simulink library "ADV_BF_MASTER"  (Simulink 8.6)
settings: Solver=VariableStepAuto  StartTime=0.0  StopTime=10.0  RelTol=1e-3
libraries: cdsEpicsOut x43, cdsFilt x36, cdsTP x20, cdsFiltCtrl x17, cdsEpicsIn x10, cdsMuxMatrix x4, VIS_LIB x2, cdsEpicsBinIn x2, cdsOsc x1, cdsFunctionCall x1, SIXOSEM_F_STAGE_MASTER x1
(part 1 of 6)
settings Model: Creator=controls  LastModifiedBy=controls

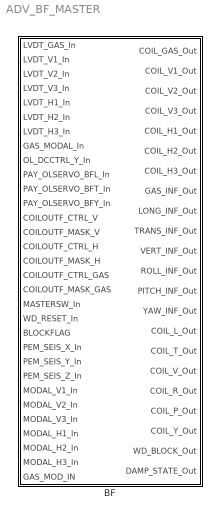
== system ADV_BF_MASTER ==
  BF : Subsystem

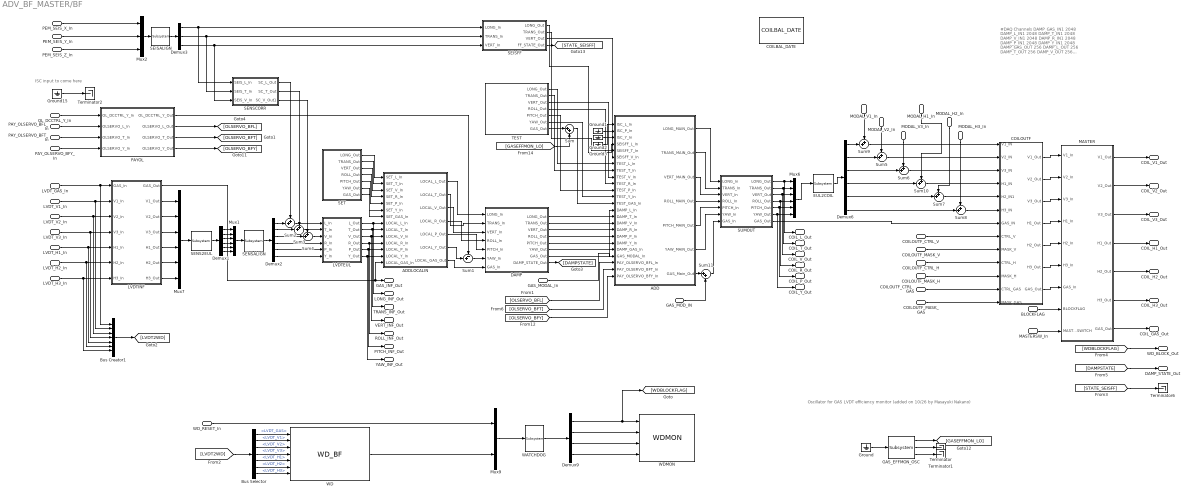
== system ADV_BF_MASTER/BF ==
  note: #DAQ Channels
      | DAMP_GAS_IN1 2048
      | DAMP_L_IN1 2048
      | DAMP_T_IN1 2048
      | DAMP_V_IN1 2048
      | DAMP_R_IN1 2048
      | DAMP_P_IN1 2048
      | DAMP_Y_IN1 2048
      | DAMP_GAS_OUT 256
      | DAMP_L_OUT 256
      | DAMP_T_OUT 256
      | DAMP_V_OUT 256
      | DAMP_R_OUT 256
      | DAMP_P_OUT 256
      | DAMP_Y_OUT 256
      | LVDTINF_GAS_IN1 2048
  note: ISC input to come here
  note: Oscillator for GAS LVDT efficiency monitor (added on 10/26 by Masayuki Nakano)
  LVDT_GAS_In : Inport
  LVDT_V1_In : Inport  Port=2
  LVDT_V2_In : Inport  Port=3
  LVDT_V3_In : Inport  Port=4
  LVDT_H1_In : Inport  Port=5
  LVDT_H2_In : Inport  Port=6
  LVDT_H3_In : Inport  Port=7
  GAS_MODAL_In : Inport  Port=8
  OL_DCCTRL_Y_In : Inport  Port=9
  PAY_OLSERVO_BFL_In : Inport  Port=10
  PAY_OLSERVO_BFT_In : Inport  Port=11
  PAY_OLSERVO_BFY_In : Inport  Port=12
  COILOUTF_CTRL_V : Inport  Port=13
  COILOUTF_MASK_V : Inport  Port=14
  COILOUTF_CTRL_H : Inport  Port=15
  COILOUTF_MASK_H : Inport  Port=16
  COILOUTF_CTRL_GAS : Inport  Port=17
  COILOUTF_MASK_GAS : Inport  Port=18
  MASTERSW_In : Inport  Port=19
  WD_RESET_In : Inport  Port=20
  BLOCKFLAG : Inport  Port=21
  PEM_SEIS_X_In : Inport  Port=22
  PEM_SEIS_Y_In : Inport  Port=23
  PEM_SEIS_Z_In : Inport  Port=24
  MODAL_V1_In : Inport  Port=25
  MODAL_V2_In : Inport  Port=26
  MODAL_V3_In : Inport  Port=27
  MODAL_H1_In : Inport  Port=28
  MODAL_H2_In : Inport  Port=29
  MODAL_H3_In : Inport  Port=30
  GAS_MOD_IN : Inport  Port=31
  ADD : Subsystem
  ADDLOCALIN : Subsystem
  Bus Creator1 : BusCreator  Inputs='LVDT_GAS','LVDT_V1','LVDT_V2','LVDT_V3','LVDT_H1','LVDT_H2','LVDT_H3'
  Bus Selector : BusSelector  OutputSignals=LVDT_GAS,LVDT_V1,LVDT_V2,LVDT_V3,LVDT_H1,LVDT_H2,LVDT_H3
  COILBAL_DATE : VIS_LIB/COILBAL_DATE
  COILOUTF : Subsystem
  DAMP : Subsystem
  Demux1 : Demux  Outputs=6
  Demux2 : Demux  Outputs=6
  Demux3 : Demux  Outputs=3
  Demux6 : Demux  Outputs=6
  Demux9 : Demux
  EUL2COIL : cdsMuxMatrix/Subsystem  Tag=cdsMuxMatrix  Description=|
      | ADL=SUS_INMATRIX.adl
      | SCRIPT=generate_KisselButton.py 4 5 #CHANNEL# > #TARGET_DIR#/#FULL_PART_NAME#_KB.adl
      settings: AttributesFormatString=%<Tag>
  GAS_EFFMON_OSC : cdsOsc/Subsystem  Tag=cdsOsc  Description=Oscillator
      settings: AttributesFormatString=%<Tag>
  Ground{,1..3,15} (5 alike) : Ground
  LVDTEUL : Subsystem
  LVDTINF : Subsystem
  MASTER : Subsystem
  Mux1 : Mux  Inputs=6
  Mux2 : Mux  Inputs=3
  Mux6 : Mux  Inputs=6
  Mux7 : Mux  Inputs=6
  Mux9 : Mux  Inputs=2
  PAYOL : Subsystem
  SEISALIGN : cdsMuxMatrix/Subsystem  Tag=cdsMuxMatrix  Description=|
      | ADL=SUS_INMATRIX.adl
      | SCRIPT=generate_KisselButton.py 4 5 #CHANNEL# > #TARGET_DIR#/#FULL_PART_NAME#_KB.adl
      settings: AttributesFormatString=%<Tag>
  SEISFF : Subsystem
  SENS2EUL : cdsMuxMatrix/Subsystem  Tag=cdsMuxMatrix  Description=Any size matrix. Inputs and outputs must be connected using Mux and Demux parts.
      settings: AttributesFormatString=%<Tag>
  SENSALIGN : cdsMuxMatrix/Subsystem  Tag=cdsMuxMatrix  Description=Any size matrix. Inputs and outputs must be connected using Mux and Demux parts.
      settings: AttributesFormatString=%<Tag>
  SENSCORR : Subsystem
  SET : Subsystem
  SUMOUT : Subsystem
  Sum : Sum  Inputs=|++
  Sum1 : Sum  Inputs=-+|
  Sum{2..10} (9 alike) : Sum  Inputs=++|
  Sum11 : Sum  Inputs=|++
  TEST : Subsystem
  Terminator{,1..2,6} (4 alike) : Terminator
  WATCHDOG : cdsFunctionCall/Subsystem  Tag=cdsFunctionCall  Description=inline OSEMWATCHDOG /opt/rtcds/userapps/release/vis/common/src/WATCHDOG.c
      settings: AttributesFormatString=%<Tag>\n%<Description>
  WD : VIS_LIB/WD_BF
  WDMON : SIXOSEM_F_STAGE_MASTER/SIXOSEM_F_STAGE_MASTER/WDMON
  COIL_GAS_Out : Outport
  COIL_V1_Out : Outport  Port=2
  COIL_V2_Out : Outport  Port=3
  COIL_V3_Out : Outport  Port=4
  COIL_H1_Out : Outport  Port=5
  COIL_H2_Out : Outport  Port=6
  COIL_H3_Out : Outport  Port=7
  GAS_INF_Out : Outport  Port=8
  LONG_INF_Out : Outport  Port=9
  TRANS_INF_Out : Outport  Port=10
  VERT_INF_Out : Outport  Port=11
  ROLL_INF_Out : Outport  Port=12
  PITCH_INF_Out : Outport  Port=13
  YAW_INF_Out : Outport  Port=14
  COIL_L_Out : Outport  Port=15
  COIL_T_Out : Outport  Port=16
  COIL_V_Out : Outport  Port=17
  COIL_R_Out : Outport  Port=18
  COIL_P_Out : Outport  Port=19
  COIL_Y_Out : Outport  Port=20
  WD_BLOCK_Out : Outport  Port=21
  DAMP_STATE_Out : Outport  Port=22
  wires:
  GAS_MOD_IN/1 -> Sum11/2
  Sum11/1 -> SUMOUT/7(GAS_In)
  ADD/7(GAS_Main_Out) -> Sum11/1
  Demux6/1 -> Sum9/2
  Demux6/6 -> Sum8/2
  MODAL_H3_In/1 -> Sum8/1
  Sum8/1 -> COILOUTF/6(H3_IN)
  Demux6/5 -> Sum7/2
  MODAL_H2_In/1 -> Sum7/1
  Sum7/1 -> COILOUTF/5(H2_IN1)
  Demux6/4 -> Sum10/2
  MODAL_H1_In/1 -> Sum10/1
  Sum10/1 -> COILOUTF/4(H1_IN)
  Demux6/3 -> Sum6/2
  MODAL_V3_In/1 -> Sum6/1
  Sum6/1 -> COILOUTF/3(V3_IN)
  Demux6/2 -> Sum5/2
  MODAL_V2_In/1 -> Sum5/1
  Sum5/1 -> COILOUTF/2(V2_IN)
  MODAL_V1_In/1 -> Sum9/1
  Sum9/1 -> COILOUTF/1(V1_IN)
  Ground15/1 -> Terminator2/1
  GAS_EFFMON_OSC/3 -> Terminator1/1
  GAS_EFFMON_OSC/2 -> Terminator/1
  Ground/1 -> GAS_EFFMON_OSC/1
  [GASEFFMON_LO] -> Sum/2
  TEST/7(GAS_Out) -> Sum/1
  GAS_EFFMON_OSC/1 -> [GASEFFMON_LO]
  COILOUTF_MASK_GAS/1 -> COILOUTF/13(MASK_GAS)
  COILOUTF_CTRL_GAS/1 -> COILOUTF/12(CTRL_GAS)
  COILOUTF_MASK_H/1 -> COILOUTF/11(MASK_H)
  COILOUTF_CTRL_H/1 -> COILOUTF/10(CTRL_H)
  LVDTINF/7(H3_Out) -> Mux7/6
  LVDTINF/6(H2_Out) -> Mux7/5
  LVDTINF/5(H1_Out) -> Mux7/4
  Bus Selector/7 -> WD/7  "<LVDT_H3>"
  Bus Selector/6 -> WD/6  "<LVDT_H2>"
  Bus Selector/5 -> WD/5  "<LVDT_H1>"
  Bus Selector/4 -> WD/4  "<LVDT_V3>"
  Bus Selector/3 -> WD/3  "<LVDT_V2>"
  Bus Selector/2 -> WD/2  "<LVDT_V1>"
  [DAMPSTATE] -> DAMP_STATE_Out/1
  [WDBLOCKFLAG] -> WD_BLOCK_Out/1
  MASTER/7(GAS_Out) -> COIL_GAS_Out/1
  MASTER/6(H3_Out) -> COIL_H3_Out/1
  MASTER/5(H2_Out) -> COIL_H2_Out/1
  MASTERSW_In/1 -> MASTER/9(MASTERSWITCH)
  BLOCKFLAG/1 -> MASTER/8(BLOCKFLAG)
  COILOUTF/4(H1_Out) -> MASTER/4(H1_In)
  COILOUTF/3(V3_Out) -> MASTER/3(V3_In)
  COILOUTF/2(V2_Out) -> MASTER/2(V2_In)
  COILOUTF/1(V1_Out) -> MASTER/1(V1_In)
  COILOUTF/7(GAS_Out) -> MASTER/7(GAS_In)
  COILOUTF/6(H3_Out) -> MASTER/6(H3_In)
  COILOUTF/5(H2_Out) -> MASTER/5(H2_In)
  DAMP/1(LONG_Out) -> ADD/14(DAMP_L_In)
  DAMP/2(TRANS_Out) -> ADD/15(DAMP_T_In)
  DAMP/3(VERT_Out) -> ADD/16(DAMP_V_In)
  DAMP/4(ROLL_Out) -> ADD/17(DAMP_R_In)
  DAMP/5(PITCH_Out) -> ADD/18(DAMP_P_In)
  DAMP/6(YAW_Out) -> ADD/19(DAMP_Y_In)
  DAMP/7(GAS_Out) -> ADD/20(DAMP_GAS_In)
  DAMP/8(DAMP_STATE_Out) -> [DAMPSTATE]
  LVDTINF/4(V3_Out) -> Mux7/3
  LVDTINF/3(V2_Out) -> Mux7/2
  LVDTINF/2(V1_Out) -> Mux7/1
  SENSALIGN/1 -> Demux2/1
  Mux1/1 -> SENSALIGN/1
  Demux1/6 -> Mux1/6
  Demux1/5 -> Mux1/5
  Demux1/4 -> Mux1/4
  Demux1/3 -> Mux1/3
  Demux1/2 -> Mux1/2
  Demux1/1 -> Mux1/1
  SENS2EUL/1 -> Demux1/1
  Bus Selector/1 -> WD/1  "<LVDT_GAS>"
  MASTER/4(H1_Out) -> COIL_H1_Out/1
  LVDT_GAS_In/1 -> LVDTINF/1(GAS_In), Bus Creator1/1
  COILOUTF_MASK_V/1 -> COILOUTF/9(MASK_V)
  COILOUTF_CTRL_V/1 -> COILOUTF/8(CTRL_V)
  Bus Creator1/1 -> [LVDT2WD]
  LVDT_H3_In/1 -> Bus Creator1/7, LVDTINF/7(H3_In)
  LVDT_H2_In/1 -> Bus Creator1/6, LVDTINF/6(H2_In)
  LVDT_H1_In/1 -> Bus Creator1/5, LVDTINF/5(H1_In)
  LVDT_V3_In/1 -> LVDTINF/4(V3_In), Bus Creator1/4
  LVDT_V2_In/1 -> LVDTINF/3(V2_In), Bus Creator1/3
  LVDT_V1_In/1 -> LVDTINF/2(V1_In), Bus Creator1/2
  WATCHDOG/1 -> Demux9/1
  Mux9/1 -> WATCHDOG/1
  Demux9/4 -> WDMON/4
  Demux9/3 -> WDMON/3
  Demux9/2 -> WDMON/2
  Demux9/1 -> WDMON/1, [WDBLOCKFLAG]
  [LVDT2WD] -> Bus Selector/1
  WD/1 -> Mux9/2
  WD_RESET_In/1 -> Mux9/1
  MASTER/3(V3_Out) -> COIL_V3_Out/1
  MASTER/2(V2_Out) -> COIL_V2_Out/1
  MASTER/1(V1_Out) -> COIL_V1_Out/1
  EUL2COIL/1 -> Demux6/1
  Mux6/1 -> EUL2COIL/1
  Mux7/1 -> SENS2EUL/1
  GAS_MODAL_In/1 -> ADD/21(GAS_MODAL_In)
  Ground1/1 -> ADD/1(ISC_L_In)
  Ground2/1 -> ADD/2(ISC_P_In)
  Ground3/1 -> ADD/3(ISC_Y_In)
  OL_DCCTRL_Y_In/1 -> PAYOL/1(OL_DCCTRL_Y_In)
  PAY_OLSERVO_BFY_In/1 -> PAYOL/4(OLSERVO_Y_In)
  PAYOL/4(OLSERVO_Y_Out) -> [OLSERVO_BFY]
  [OLSERVO_BFY] -> ADD/24(PAY_OLSERVO_BFY_In)
  SEISFF/4(FF_STATE_Out) -> [STATE_SEISFF]
  PEM_SEIS_Y_In/1 -> Mux2/2
  PEM_SEIS_X_In/1 -> Mux2/1
  Mux2/1 -> SEISALIGN/1
  SEISALIGN/1 -> Demux3/1
  Demux3/2 -> SEISFF/2(TRANS_In), SENSCORR/2(SEIS_T_In)
  Demux3/1 -> SEISFF/1(LONG_In), SENSCORR/1(SEIS_L_In)
  PEM_SEIS_Z_In/1 -> Mux2/3
  Demux3/3 -> SEISFF/3(VERT_In), SENSCORR/3(SEIS_V_In)
  SENSCORR/1(SC_L_Out) -> Sum2/1
  SENSCORR/2(SC_T_Out) -> Sum3/1
  SENSCORR/3(SC_V_Out1) -> Sum4/1
  Demux2/1 -> Sum2/2
  Demux2/2 -> Sum3/2
  Demux2/3 -> Sum4/2
  TEST/1(LONG_Out) -> ADD/7(TEST_L_In)
  TEST/2(TRANS_Out) -> ADD/8(TEST_T_In)
  TEST/3(VERT_Out) -> ADD/9(TEST_V_In)
  TEST/4(ROLL_Out) -> ADD/10(TEST_R_In)
  TEST/5(PITCH_Out) -> ADD/11(TEST_P_In)
  TEST/6(YAW_Out) -> ADD/12(TEST_Y_In)
  Sum/1 -> ADD/13(TEST_GAS_In)
  [STATE_SEISFF] -> Terminator6/1
  SEISFF/3(VERT_Out) -> ADD/6(SEISFF_V_In)
  SEISFF/1(LONG_Out) -> ADD/4(SEISFF_L_In)
  SEISFF/2(TRANS_Out) -> ADD/5(SEISFF_T_In)
  Sum2/1 -> LVDTEUL/1(L_In)
  Sum3/1 -> LVDTEUL/2(T_In)
  Sum4/1 -> LVDTEUL/3(V_In)
  Demux2/4 -> LVDTEUL/4(R_In)
  Demux2/5 -> LVDTEUL/5(P_In)
  Demux2/6 -> LVDTEUL/6(Y_In)
  SET/2(TRANS_Out) -> ADDLOCALIN/2(SET_T_In)
  SET/3(VERT_Out) -> ADDLOCALIN/3(SET_V_In)
  SET/7(GAS_Out) -> ADDLOCALIN/7(SET_GAS_In)
  SET/5(PITCH_Out) -> ADDLOCALIN/5(SET_P_In)
  SET/1(LONG_Out) -> ADDLOCALIN/1(SET_L_In)
  SET/4(ROLL_Out) -> ADDLOCALIN/4(SET_R_In)
  SET/6(YAW_Out) -> ADDLOCALIN/6(SET_Y_In)
  LVDTEUL/6(Y_Out) -> YAW_INF_Out/1, ADDLOCALIN/13(LOCAL_Y_In)
  LVDTEUL/1(L_Out) -> LONG_INF_Out/1, ADDLOCALIN/8(LOCAL_L_In)
  LVDTEUL/2(T_Out) -> TRANS_INF_Out/1, ADDLOCALIN/9(LOCAL_T_In)
  LVDTEUL/3(V_Out) -> VERT_INF_Out/1, ADDLOCALIN/10(LOCAL_V_In)
  LVDTEUL/4(R_Out) -> ROLL_INF_Out/1, ADDLOCALIN/11(LOCAL_R_In)
  LVDTEUL/5(P_Out) -> PITCH_INF_Out/1, ADDLOCALIN/12(LOCAL_P_In)
  ADDLOCALIN/7(LOCAL_GAS_Out) -> DAMP/7(GAS_In)
  ADDLOCALIN/6(LOCAL_Y_Out) -> Sum1/2
  ADDLOCALIN/5(LOCAL_P_Out) -> DAMP/5(PITCH_In)
  ADDLOCALIN/4(LOCAL_R_Out) -> DAMP/4(ROLL_In)
  ADDLOCALIN/3(LOCAL_V_Out) -> DAMP/3(VERT_In)
  ADDLOCALIN/2(LOCAL_T_Out) -> DAMP/2(TRANS_In)
  ADDLOCALIN/1(LOCAL_L_Out) -> DAMP/1(LONG_In)
  LVDTINF/1(GAS_Out) -> GAS_INF_Out/1, ADDLOCALIN/14(LOCAL_GAS_In)
  Sum1/1 -> DAMP/6(YAW_In)
  PAYOL/1(OL_DCCTRL_Y_Out) -> Sum1/1
  [OLSERVO_BFL] -> ADD/22(PAY_OLSERVO_BFL_In)
  [OLSERVO_BFT] -> ADD/23(PAY_OLSERVO_BFT_In)
  PAY_OLSERVO_BFL_In/1 -> PAYOL/2(OLSERVO_L_In)
  PAY_OLSERVO_BFT_In/1 -> PAYOL/3(OLSERVO_T_In)
  PAYOL/3(OLSERVO_T_Out) -> [OLSERVO_BFT]
  PAYOL/2(OLSERVO_L_Out) -> [OLSERVO_BFL]
  SUMOUT/1(LONG_Out) -> COIL_L_Out/1, Mux6/1
  SUMOUT/6(YAW_Out) -> COIL_Y_Out/1, Mux6/6
  SUMOUT/3(VERT_Out) -> COIL_V_Out/1, Mux6/3
  SUMOUT/2(TRANS_Out) -> COIL_T_Out/1, Mux6/2
  SUMOUT/4(ROLL_Out) -> COIL_R_Out/1, Mux6/4
  SUMOUT/5(PITCH_Out) -> COIL_P_Out/1, Mux6/5
  SUMOUT/7(GAS_Out) -> COILOUTF/7(GAS_IN)
  ADD/4(ROLL_MAIN_Out) -> SUMOUT/4(ROLL_In)
  ADD/3(VERT_MAIN_Out) -> SUMOUT/3(VERT_In)
  ADD/5(PITCH_MAIN_Out) -> SUMOUT/5(PITCH_In)
  ADD/2(TRANS_MAIN_Out) -> SUMOUT/2(TRANS_In)
  ADD/6(YAW_MAIN_Out) -> SUMOUT/6(YAW_In)
  ADD/1(LONG_MAIN_Out) -> SUMOUT/1(LONG_In)

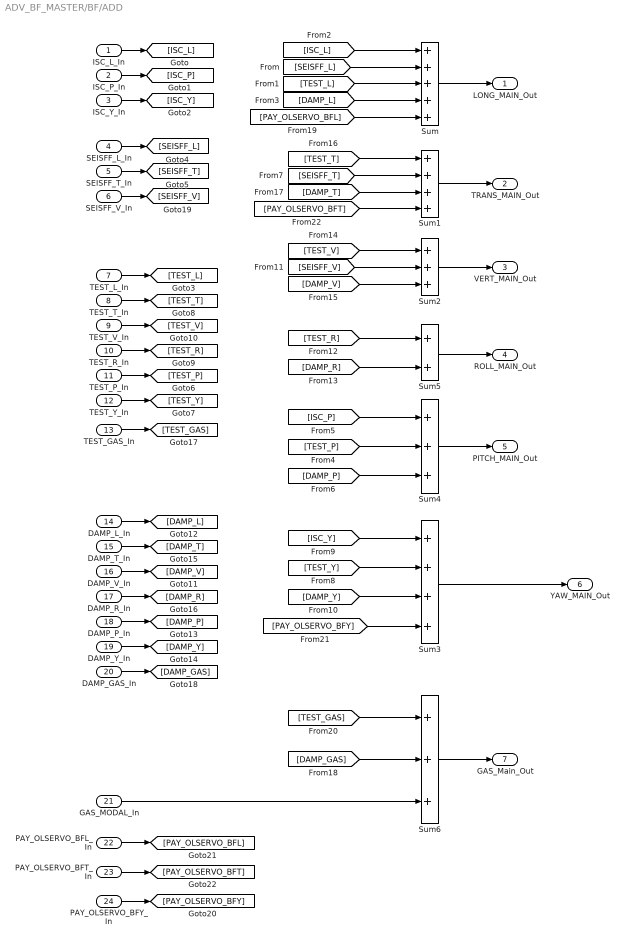
== system ADV_BF_MASTER/BF/ADD ==
  ISC_L_In : Inport
  ISC_P_In : Inport  Port=2
  ISC_Y_In : Inport  Port=3
  SEISFF_L_In : Inport  Port=4
  SEISFF_T_In : Inport  Port=5
  SEISFF_V_In : Inport  Port=6
  TEST_L_In : Inport  Port=7
  TEST_T_In : Inport  Port=8
  TEST_V_In : Inport  Port=9
  TEST_R_In : Inport  Port=10
  TEST_P_In : Inport  Port=11
  TEST_Y_In : Inport  Port=12
  TEST_GAS_In : Inport  Port=13
  DAMP_L_In : Inport  Port=14
  DAMP_T_In : Inport  Port=15
  DAMP_V_In : Inport  Port=16
  DAMP_R_In : Inport  Port=17
  DAMP_P_In : Inport  Port=18
  DAMP_Y_In : Inport  Port=19
  DAMP_GAS_In : Inport  Port=20
  GAS_MODAL_In : Inport  Port=21
  PAY_OLSERVO_BFL_In : Inport  Port=22
  PAY_OLSERVO_BFT_In : Inport  Port=23
  PAY_OLSERVO_BFY_In : Inport  Port=24
  Sum : Sum  Inputs=+++++
  Sum1 : Sum  Inputs=++++
  Sum2 : Sum  Inputs=+++
  Sum3 : Sum  Inputs=++++
  Sum4 : Sum  Inputs=+++
  Sum5 : Sum
  Sum6 : Sum  Inputs=+++
  LONG_MAIN_Out : Outport
  TRANS_MAIN_Out : Outport  Port=2
  VERT_MAIN_Out : Outport  Port=3
  ROLL_MAIN_Out : Outport  Port=4
  PITCH_MAIN_Out : Outport  Port=5
  YAW_MAIN_Out : Outport  Port=6
  GAS_Main_Out : Outport  Port=7
  wires:
  DAMP_GAS_In/1 -> [DAMP_GAS]
  DAMP_Y_In/1 -> [DAMP_Y]
  DAMP_P_In/1 -> [DAMP_P]
  DAMP_R_In/1 -> [DAMP_R]
  DAMP_V_In/1 -> [DAMP_V]
  DAMP_T_In/1 -> [DAMP_T]
  DAMP_L_In/1 -> [DAMP_L]
  TEST_GAS_In/1 -> [TEST_GAS]
  TEST_Y_In/1 -> [TEST_Y]
  TEST_P_In/1 -> [TEST_P]
  TEST_R_In/1 -> [TEST_R]
  TEST_V_In/1 -> [TEST_V]
  TEST_T_In/1 -> [TEST_T]
  TEST_L_In/1 -> [TEST_L]
  SEISFF_V_In/1 -> [SEISFF_V]
  Sum6/1 -> GAS_Main_Out/1
  Sum4/1 -> PITCH_MAIN_Out/1
  Sum/1 -> LONG_MAIN_Out/1
  [ISC_L] -> Sum/1
  [TEST_L] -> Sum/3
  [DAMP_L] -> Sum/4
  Sum5/1 -> ROLL_MAIN_Out/1
  Sum2/1 -> VERT_MAIN_Out/1
  Sum1/1 -> TRANS_MAIN_Out/1
  SEISFF_L_In/1 -> [SEISFF_L]
  SEISFF_T_In/1 -> [SEISFF_T]
  ISC_L_In/1 -> [ISC_L]
  ISC_P_In/1 -> [ISC_P]
  ISC_Y_In/1 -> [ISC_Y]
  [ISC_P] -> Sum4/1
  [TEST_R] -> Sum5/1
  [DAMP_R] -> Sum5/2
  [TEST_T] -> Sum1/1
  [DAMP_T] -> Sum1/3
  [TEST_V] -> Sum2/1
  [DAMP_V] -> Sum2/3
  PAY_OLSERVO_BFY_In/1 -> [PAY_OLSERVO_BFY]
  Sum3/1 -> YAW_MAIN_Out/1
  [SEISFF_L] -> Sum/2
  [SEISFF_T] -> Sum1/2
  [SEISFF_V] -> Sum2/2
  [TEST_P] -> Sum4/2
  [DAMP_P] -> Sum4/3
  [PAY_OLSERVO_BFY] -> Sum3/4
  [DAMP_Y] -> Sum3/3
  [TEST_Y] -> Sum3/2
  [ISC_Y] -> Sum3/1
  [TEST_GAS] -> Sum6/1
  [DAMP_GAS] -> Sum6/2
  GAS_MODAL_In/1 -> Sum6/3
  PAY_OLSERVO_BFL_In/1 -> [PAY_OLSERVO_BFL]
  PAY_OLSERVO_BFT_In/1 -> [PAY_OLSERVO_BFT]
  [PAY_OLSERVO_BFL] -> Sum/5
  [PAY_OLSERVO_BFT] -> Sum1/4

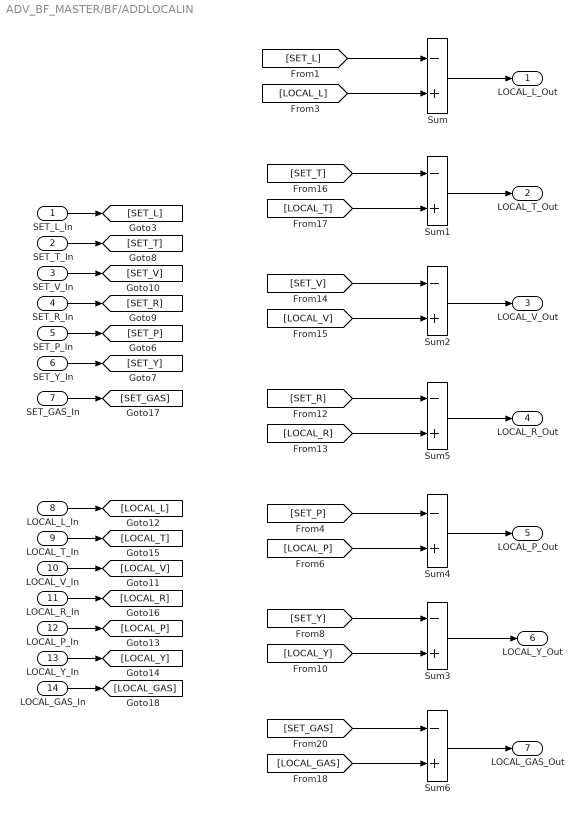
== system ADV_BF_MASTER/BF/ADDLOCALIN ==
  SET_L_In : Inport
  SET_T_In : Inport  Port=2
  SET_V_In : Inport  Port=3
  SET_R_In : Inport  Port=4
  SET_P_In : Inport  Port=5
  SET_Y_In : Inport  Port=6
  SET_GAS_In : Inport  Port=7
  LOCAL_L_In : Inport  Port=8
  LOCAL_T_In : Inport  Port=9
  LOCAL_V_In : Inport  Port=10
  LOCAL_R_In : Inport  Port=11
  LOCAL_P_In : Inport  Port=12
  LOCAL_Y_In : Inport  Port=13
  LOCAL_GAS_In : Inport  Port=14
  Sum{,1..6} (7 alike) : Sum  Inputs=-+
  LOCAL_L_Out : Outport
  LOCAL_T_Out : Outport  Port=2
  LOCAL_V_Out : Outport  Port=3
  LOCAL_R_Out : Outport  Port=4
  LOCAL_P_Out : Outport  Port=5
  LOCAL_Y_Out : Outport  Port=6
  LOCAL_GAS_Out : Outport  Port=7
  wires:
  LOCAL_GAS_In/1 -> [LOCAL_GAS]
  LOCAL_Y_In/1 -> [LOCAL_Y]
  LOCAL_P_In/1 -> [LOCAL_P]
  LOCAL_R_In/1 -> [LOCAL_R]
  LOCAL_V_In/1 -> [LOCAL_V]
  LOCAL_T_In/1 -> [LOCAL_T]
  LOCAL_L_In/1 -> [LOCAL_L]
  SET_GAS_In/1 -> [SET_GAS]
  SET_Y_In/1 -> [SET_Y]
  SET_P_In/1 -> [SET_P]
  SET_R_In/1 -> [SET_R]
  SET_V_In/1 -> [SET_V]
  SET_T_In/1 -> [SET_T]
  SET_L_In/1 -> [SET_L]
  Sum6/1 -> LOCAL_GAS_Out/1
  Sum4/1 -> LOCAL_P_Out/1
  Sum/1 -> LOCAL_L_Out/1
  Sum5/1 -> LOCAL_R_Out/1
  Sum2/1 -> LOCAL_V_Out/1
  Sum1/1 -> LOCAL_T_Out/1
  Sum3/1 -> LOCAL_Y_Out/1
  [SET_L] -> Sum/1
  [LOCAL_L] -> Sum/2
  [LOCAL_T] -> Sum1/2
  [SET_T] -> Sum1/1
  [LOCAL_V] -> Sum2/2
  [SET_V] -> Sum2/1
  [LOCAL_R] -> Sum5/2
  [SET_R] -> Sum5/1
  [LOCAL_P] -> Sum4/2
  [SET_P] -> Sum4/1
  [LOCAL_Y] -> Sum3/2
  [SET_Y] -> Sum3/1
  [SET_GAS] -> Sum6/1
  [LOCAL_GAS] -> Sum6/2
